simulink model "model"  (R2024a)
settings: Solver=VariableStepAuto  StartTime=0.0  StopTime=simulation_time  RelTol=1e-3
values from neighbouring files (symbols this model uses):
  ddq_d = @(t) (delta_q/simulation_time^2).*(6*a*(t/simulation_time) + 2*b)    [example.m]
  dq_0 = zeros(n, 1)    [example.m]
  dq_d = @(t) (delta_q/simulation_time).*(3*a*(t/simulation_time)^2 + 2*b*(t/simulation_time) + c)    [example.m]
  q_0 = randn(n, 1)    [example.m]
  q_d = @(t) q_d_start + delta_q.*(a*(t/simulation_time)^3 + b*(t/simulation_time)^2 + c*t/simulation_time)    [example.m]
libraries: robotmaniplib x2
settings Model: Creator=pietro  LastModifiedBy=pietro

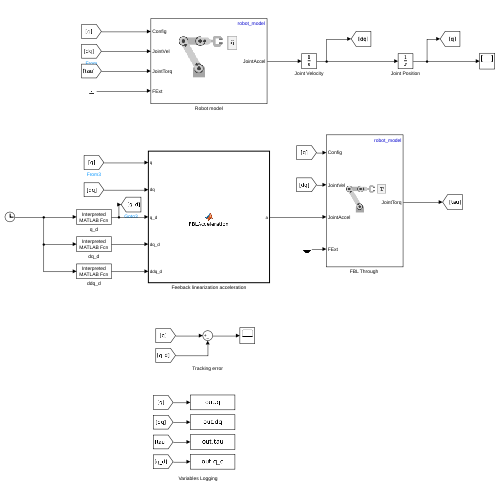
[thumbnail: Simulink's stored preview of the top-level diagram]
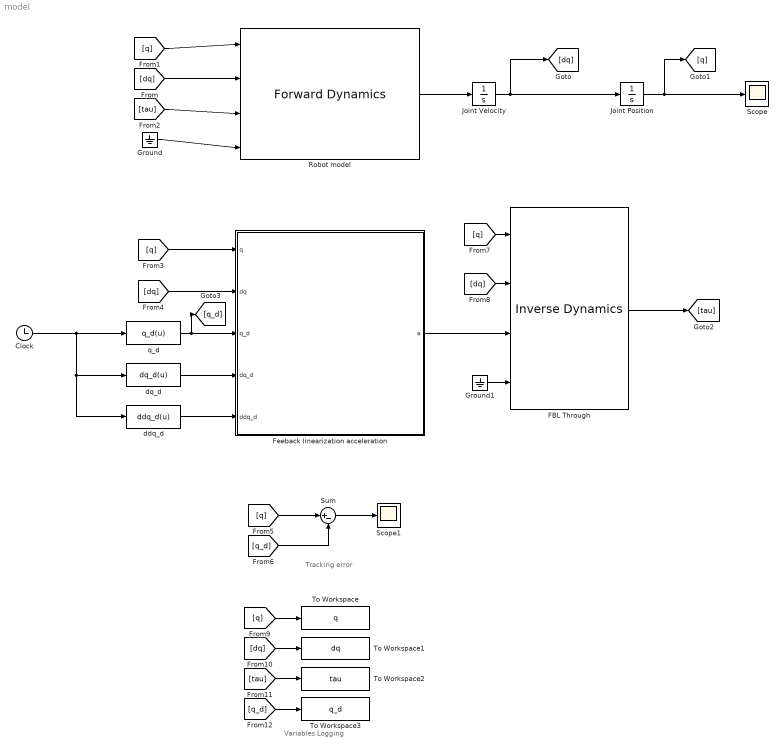
== system model ==
  note: Variables Logging
  note: Tracking error
  Clock : Clock
  "FBL Through " : robotmaniplib/Inverse Dynamics  RigidBodyTree=robot_model  SimulateUsing=Code generation
  Feeback linearization acceleration : MATLAB Function  TreatAsAtomicUnit=on
  Ground : Ground
  Ground1 : Ground
  Joint Position : Integrator  InitialCondition=q_0
  Joint Velocity : Integrator  InitialCondition=dq_0
  Robot model : robotmaniplib/Forward Dynamics  RigidBodyTree=robot_model  SimulateUsing=Code generation
  Scope : Scope
  Scope1 : Scope
  Sum : Sum  Inputs=|+-
  To Workspace : ToWorkspace  VariableName=q  SaveFormat=Timeseries  SampleTime=-1
  To Workspace1 : ToWorkspace  VariableName=dq  SaveFormat=Timeseries  SampleTime=-1
  To Workspace2 : ToWorkspace  VariableName=tau  SaveFormat=Timeseries  SampleTime=-1
  To Workspace3 : ToWorkspace  VariableName=q_d  SaveFormat=Timeseries  SampleTime=-1
  ddq_d : MATLABFcn  MATLABFcn=ddq_d(u)
  dq_d : MATLABFcn  MATLABFcn=dq_d(u)
  q_d : MATLABFcn  MATLABFcn=q_d(u)
  wires:
  Robot model/1 -> Joint Velocity/1
  Joint Velocity/1 -> [dq], Joint Position/1
  [dq] -> Robot model/2
  Joint Position/1 -> Scope/1, [q]
  [q] -> Robot model/1
  [tau] -> Robot model/3
  Ground/1 -> Robot model/4
  [q] -> Feeback linearization acceleration/1(q)
  [dq] -> Feeback linearization acceleration/2(dq)
  q_d/1 -> [q_d], Feeback linearization acceleration/3(q_d)
  Clock/1 -> ddq_d/1, dq_d/1, q_d/1
  dq_d/1 -> Feeback linearization acceleration/4(dq_d)
  ddq_d/1 -> Feeback linearization acceleration/5(ddq_d)
  [q] -> Sum/1
  [q_d] -> Sum/2
  Sum/1 -> Scope1/1
  "FBL Through "/1 -> [tau]
  Feeback linearization acceleration/1(a) -> "FBL Through "/3
  [q] -> "FBL Through "/1
  [dq] -> "FBL Through "/2
  Ground1/1 -> "FBL Through "/4
  [q] -> To Workspace/1
  [dq] -> To Workspace1/1
  [tau] -> To Workspace2/1
  [q_d] -> To Workspace3/1

== matlab function model/Feeback linearization acceleration ==
  data: q input; a output; dq input; q_d input; dq_d input; ddq_d input
function a = FBLAcceleration(q, dq, q_d, dq_d, ddq_d)

% Control gains
K_P = 100;
K_D = 10;

% Acceleration command of the FBL controller
a   = ddq_d + K_P*(q_d - q) + K_D*(dq_d - dq);

end
